simulink model "slinkprovadeconceito"  (R2015a)
settings: Solver=ode45  StartTime=0.0  StopTime=10.0  RelTol=1e-3
libraries: simulink x1
settings Model: Creator=user  LastModifiedBy=user

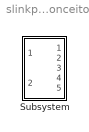
== system slinkprovadeconceito ==
  Subsystem : Subsystem

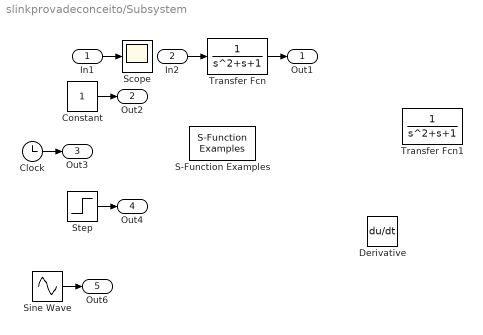
== system slinkprovadeconceito/Subsystem ==
  In1 : Inport
  In2 : Inport  Port=2
  Clock : Clock
  Constant : Constant
  Derivative : Derivative
  S-Function Examples : simulink/User-Defined Functions/S-Function Examples
  Scope : Scope
  Sine Wave : Sin  SampleTime=0
  Step : Step  SampleTime=0
  Transfer Fcn : TransferFcn  Denominator=[1 1 1]
  Transfer Fcn1 : TransferFcn  Denominator=[1 1 1]
  Out1 : Outport
  Out2 : Outport  Port=2
  Out3 : Outport  Port=3
  Out4 : Outport  Port=4
  Out6 : Outport  Port=5
  wires:
  In1/1 -> Scope/1
  Clock/1 -> Out3/1
  Sine Wave/1 -> Out6/1
  In2/1 -> Transfer Fcn/1
  Transfer Fcn/1 -> Out1/1
  Step/1 -> Out4/1
  Constant/1 -> Out2/1
